simulink library "csc_vlm_valve_manager_lib"  (R2014b)
settings: Solver=ode45  StartTime=0.0  StopTime=10.0  RelTol=1e-3
libraries: util_common_lib x5, csu_pvs_pressurant_valve_switch_lib x4, util_info_lib x1
settings Model: Creator=escrane  LastModifiedBy=mstewart

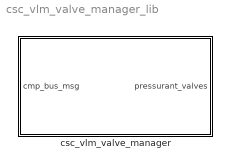
== system csc_vlm_valve_manager_lib ==
  " csc_vlm_valve_manager" : Subsystem

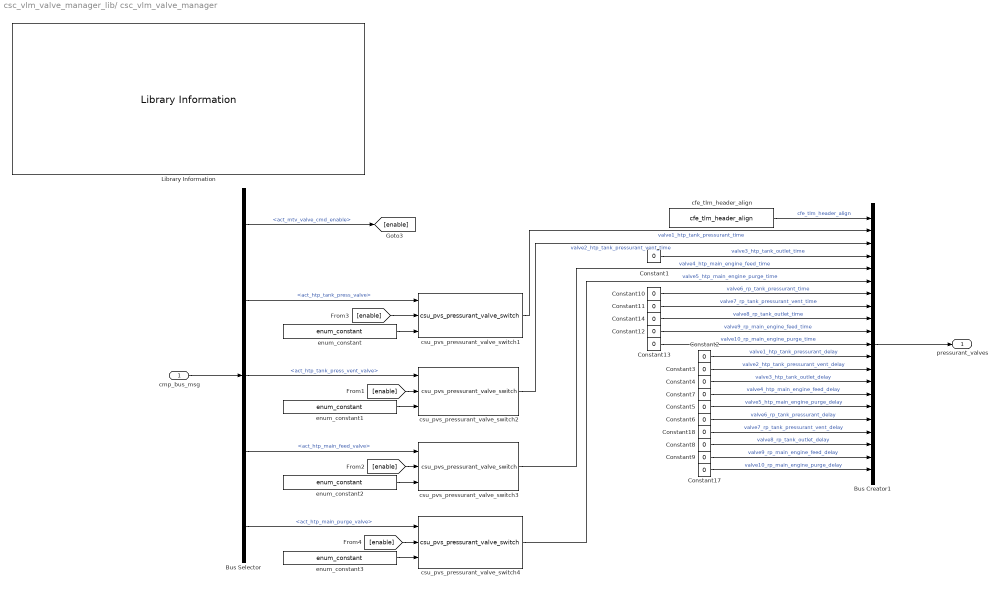
== system csc_vlm_valve_manager_lib/ csc_vlm_valve_manager ==
  cmp_bus_msg : Inport
  Bus Creator1 : BusCreator  Inputs=21
  Bus Selector : BusSelector  OutputSignals=act_mtv_valve_cmd_enable,act_htp_tank_press_valve,act_htp_tank_press_vent_valve,act_htp_main_feed_valve,act_htp_main_purge_valve
  Constant{1..14,17..18} (16 alike) : Constant  Value=0  OutDataTypeStr=uint8
  Library Information : util_info_lib/Library Information  owner='escrane'
  cfe_tlm_header_align : util_common_lib/cfe_tlm_header_align
  csu_pvs_pressurant_valve_switch1 : csu_pvs_pressurant_valve_switch_lib/csu_pvs_pressurant_valve_switch  open_duration=act_full_on_duration  closed_duration=0  event_id=22
  csu_pvs_pressurant_valve_switch2 : csu_pvs_pressurant_valve_switch_lib/csu_pvs_pressurant_valve_switch  open_duration=0  closed_duration=act_full_on_duration  event_id=23
  csu_pvs_pressurant_valve_switch3 : csu_pvs_pressurant_valve_switch_lib/csu_pvs_pressurant_valve_switch  open_duration=act_full_on_duration  closed_duration=0  event_id=24
  csu_pvs_pressurant_valve_switch4 : csu_pvs_pressurant_valve_switch_lib/csu_pvs_pressurant_valve_switch  open_duration=act_full_on_duration  closed_duration=0  event_id=25
  enum_constant{,1..3} (4 alike) : util_common_lib/enum_constant
  pressurant_valves : Outport
  wires:
  enum_constant3/1 -> csu_pvs_pressurant_valve_switch4/3
  enum_constant2/1 -> csu_pvs_pressurant_valve_switch3/3
  enum_constant1/1 -> csu_pvs_pressurant_valve_switch2/3
  enum_constant/1 -> csu_pvs_pressurant_valve_switch1/3
  Bus Selector/5 -> csu_pvs_pressurant_valve_switch4/1  "<act_htp_main_purge_valve>"
  Bus Selector/4 -> csu_pvs_pressurant_valve_switch3/1  "<act_htp_main_feed_valve>"
  Bus Selector/3 -> csu_pvs_pressurant_valve_switch2/1  "<act_htp_tank_press_vent_valve>"
  [enable] -> csu_pvs_pressurant_valve_switch4/2
  [enable] -> csu_pvs_pressurant_valve_switch3/2
  [enable] -> csu_pvs_pressurant_valve_switch2/2
  Constant2/1 -> Bus Creator1/12  "valve1_htp_tank_pressurant_delay"
  Constant8/1 -> Bus Creator1/19  "valve8_rp_tank_outlet_delay"
  Constant9/1 -> Bus Creator1/20  "valve9_rp_main_engine_feed_delay"
  Constant18/1 -> Bus Creator1/18  "valve7_rp_tank_pressurant_vent_delay"
  Constant7/1 -> Bus Creator1/15  "valve4_htp_main_engine_feed_delay"
  Constant6/1 -> Bus Creator1/17  "valve6_rp_tank_pressurant_delay"
  Constant4/1 -> Bus Creator1/14  "valve3_htp_tank_outlet_delay"
  Constant5/1 -> Bus Creator1/16  "valve5_htp_main_engine_purge_delay"
  Constant17/1 -> Bus Creator1/21  "valve10_rp_main_engine_purge_delay"
  Constant3/1 -> Bus Creator1/13  "valve2_htp_tank_pressurant_vent_delay"
  Bus Selector/2 -> csu_pvs_pressurant_valve_switch1/1  "<act_htp_tank_press_valve>"
  [enable] -> csu_pvs_pressurant_valve_switch1/2
  Bus Selector/1 -> [enable]  "<act_mtv_valve_cmd_enable>"
  Bus Creator1/1 -> pressurant_valves/1
  cfe_tlm_header_align/1 -> Bus Creator1/1  "cfe_tlm_header_align"
  csu_pvs_pressurant_valve_switch1/1 -> Bus Creator1/2  "valve1_htp_tank_pressurant_time"
  Constant14/1 -> Bus Creator1/9  "valve8_rp_tank_outlet_time"
  Constant12/1 -> Bus Creator1/10  "valve9_rp_main_engine_feed_time"
  Constant11/1 -> Bus Creator1/8  "valve7_rp_tank_pressurant_vent_time"
  csu_pvs_pressurant_valve_switch3/1 -> Bus Creator1/5  "valve4_htp_main_engine_feed_time"
  Constant10/1 -> Bus Creator1/7  "valve6_rp_tank_pressurant_time"
  Constant1/1 -> Bus Creator1/4  "valve3_htp_tank_outlet_time"
  csu_pvs_pressurant_valve_switch4/1 -> Bus Creator1/6  "valve5_htp_main_engine_purge_time"
  Constant13/1 -> Bus Creator1/11  "valve10_rp_main_engine_purge_time"
  csu_pvs_pressurant_valve_switch2/1 -> Bus Creator1/3  "valve2_htp_tank_pressurant_vent_time"
  cmp_bus_msg/1 -> Bus Selector/1
